simulink model "model_tmp_4p"  (R2015b)
settings: Solver=ode45  StartTime=0.0  StopTime=T_sim  FixedStep=dt  RelTol=1e-3
PreLoadFcn:
  | setup_tmp_4p;
InitFcn:
  | setup_tmp_4p;
StartFcn:
  | setup_tmp_4p;
values from neighbouring files (symbols this model uses):
  A_act = [-100 0 0 0 0 -100 0 0 0 0 -100 0 ... (16 elements, 4x4)]    [CD_spline.mat]    (also in CL_spline.mat; setup.m = -100*eye(4); setup_tmp_1p.m = -100*eye(4); setup_tmp_4p.m = -100*eye(4))
  A_init = [1.0386 0 12.9]    [CD_spline.mat]    (also in CL_spline.mat; setup_KiteModel_4points.m = Pc_init + d_n_r * w_k * w_rel * [-1;0;0])
  A_Kite = 7    [CD_spline.mat]    (also in CL_spline.mat; setup.m = 10.18; setup_tmp_1p.m = 10.18; setup_tmp_4p.m = 10.18)
  A_prd = [0 0 0 -640 0 0 0 0 0 0 -640 0 ... (36 elements, 6x6)]    [CD_spline.mat]    (also in CL_spline.mat; setup.m = 1000 * A_M_aug; setup_tmp_1p.m = 1000 * A_M_aug; setup_tmp_4p.m = 1000 * A_M_aug)
  A_ref = [0 0 0 -10000 0 0 0 0 0 0 -10000 0 ... (36 elements, 6x6)]    [CD_spline.mat]    (also in CL_spline.mat; setup.m = zeros(6); setup_tmp_1p.m = zeros(6); setup_tmp_4p.m = zeros(6))
  A_t_ref_cl = [0 0 0 -0.64 0 0 0 0 0 0 -0.64 0 ... (36 elements, 6x6)]    [CD_spline.mat]    (also in CL_spline.mat; setup.m = A_t_ref; setup_tmp_1p.m = A_t_ref; setup_tmp_4p.m = A_t_ref)
  alpha_0 = 10 * pi/180    (= 0.174532925199)    [setup_KiteModel_4points.m]
  alpha_d_max = 31 * pi/180    (= 0.541052068118)    [setup_KiteModel_4points.m]
  alpha_s_0 = 10 * pi/180    (= 0.174532925199)    [setup_KiteModel_4points.m]
  alpha_s_max = 20 * pi/180    (= 0.349065850399)    [setup_KiteModel_4points.m]
  ASideRel = 0    [CD_spline.mat]    (also in CL_spline.mat; setup.m; setup_tmp_1p.m; setup_tmp_4p.m = 0.306)
  B_act = [100 0 0 0 0 100 0 0 0 0 100 0 ... (16 elements, 4x4)]    [CD_spline.mat]    (also in CL_spline.mat; setup.m = 100*eye(4); setup_tmp_1p.m = 100*eye(4); setup_tmp_4p.m = 100*eye(4))
  B_init = [0 0 15.13]    [CD_spline.mat]    (also in CL_spline.mat; setup_KiteModel_4points.m = Pc_init + h_kite * [0;0;1;])
  B_ref = [0 0 0 10000 0 0 0 0 0 0 10000 0 ... (18 elements, 6x3)]    [CD_spline.mat]    (also in CL_spline.mat; setup.m = zeros(6,3); setup_tmp_1p.m = zeros(6,3); setup_tmp_4p.m = zeros(6,3))
  B_t_ref_cl = [0 0 0 0.64 0 0 0 0 0 0 0.64 0 ... (18 elements, 6x3)]    [CD_spline.mat]    (also in CL_spline.mat)
  Bpbl = [0 0 0 1 0 0 0 0 0 0 1 0 ... (18 elements, 6x3)]    [CD_spline.mat]    (also in CL_spline.mat; setup.m = [zeros(3); eye(3)]; setup_tmp_1p.m = [zeros(3); eye(3)]; setup_tmp_4p.m = [zeros(3); eye(3)])
  c0 = 614000    [CD_spline.mat]    (also in CL_spline.mat; setup.m; setup_tmp_1p.m; setup_tmp_4p.m)
  c_1_TR = 0.262    [setup_KiteModel_4points.m]
  C_A = [0 0.3 -1e-06 1 -0.3 0 1e-06 1 0 -0.3 -1e-06 1 ... (16 elements, 4x4)]    [CD_spline.mat]    (also in CL_spline.mat; setup.m = [0, -R, 0, R; setup_tmp_1p.m = [0, -R, 0, R; setup_tmp_4p.m = [0, -R, 0, R)
  C_A_inv = [0 -1.66666666667 -1.23358113847e-17 1.66666666667 1.66666666667 2.46716227694e-17 -1.66666666667 0 -250000 250000 -250000 250000 ... (16 elements, 4x4)]    [CD_spline.mat]    (also in CL_spline.mat; setup.m = C_A \eye(4); setup_tmp_1p.m = C_A \eye(4); setup_tmp_4p.m = C_A \eye(4))
  C_init = [0 2.5965 12.9]    [CD_spline.mat]    (also in CL_spline.mat; setup_KiteModel_4points.m = Pc_init + 0.5 * w_k * w_rel * [0;1;0])
  CD_spline_coefs = CD_spline.coefs    [setup_KiteModel_4points.m]
  CD_tether = 0.96    [CD_spline.mat]    (also in CL_spline.mat; setup.m; setup_tmp_1p.m; setup_tmp_4p.m)
  CL_spline_coefs = CL_spline.coefs    [setup_KiteModel_4points.m]
  d0 = 473    [CD_spline.mat]    (also in CL_spline.mat; setup.m; setup_tmp_1p.m; setup_tmp_4p.m)
  D_init = [0 -2.5965 12.9]    [CD_spline.mat]    (also in CL_spline.mat; setup_KiteModel_4points.m = Pc_init - 0.5 * w_k * w_rel * [0;1;0])
  d_tether = 0.004    [CD_spline.mat]    (also in CL_spline.mat; setup.m; setup_tmp_1p.m; setup_tmp_4p.m)
  delta_dead = 0.5    [CD_spline.mat]    (also in CL_spline.mat; setup.m; setup_tmp_1p.m; setup_tmp_4p.m)
  e_0 = 0.01    [CD_spline.mat]    (also in CL_spline.mat; setup.m; setup_tmp_1p.m; setup_tmp_4p.m)
  epsilon = 0.6    [CD_spline.mat]    (also in CL_spline.mat; setup.m; setup_tmp_1p.m; setup_tmp_4p.m)
  g = 9.81    [CD_spline.mat]    (also in CL_spline.mat; setup.m; setup_tmp_1p.m; setup_tmp_4p.m)
  g_vec = [0 0 9.81]    [CD_spline.mat]    (also in CL_spline.mat; setup.m = [0;0;9.81]; setup_tmp_1p.m = [0;0;9.81]; setup_tmp_4p.m = [0;0;9.81])
  Gamma_ad = 100    [CD_spline.mat]    (also in CL_spline.mat; setup.m = 100;100; setup_tmp_1p.m = 100;100; setup_tmp_4p.m = 100;100)
  Gamma_pred = 100    [CD_spline.mat]    (also in CL_spline.mat; setup.m; setup_tmp_1p.m; setup_tmp_4p.m)
  J = [0.018  0  0; 0  0.018  0; 0  0  0.009]    [CD_spline.mat]    (also in CL_spline.mat; setup.m = diag([Ixx, Iyy, Izz]); setup_tmp_1p.m = diag([Ixx, Iyy, Izz]); setup_tmp_4p.m = diag([Ixx, Iyy, Izz]))
  Jinv = [55.5555555556  0  0; 0  55.5555555556  0; 0  0  111.111111111]    [CD_spline.mat]    (also in CL_spline.mat; setup.m = J \ eye(3); setup_tmp_1p.m = J \ eye(3); setup_tmp_4p.m = J \ eye(3))
  K = 1 - ASideRel    [setup_KiteModel_4points.m]
  K_d_s = 1.5    [setup_KiteModel_4points.m]
  k_e_eta = 10000    [CD_spline.mat]    (also in CL_spline.mat; setup.m; setup_tmp_1p.m; setup_tmp_4p.m)
  k_e_eta_dot = 400    [CD_spline.mat]    (also in CL_spline.mat; setup.m; setup_tmp_1p.m; setup_tmp_4p.m)
  k_e_eta_I = 1    [CD_spline.mat]    (also in CL_spline.mat; setup.m; setup_tmp_1p.m; setup_tmp_4p.m)
  K_e_psi = 10    [setup_tmp_4p.m]
  K_i_t = [10  0  0; 0  10  0; 0  0  10]    [CD_spline.mat]    (also in CL_spline.mat; setup.m = 10*eye(3); setup_tmp_1p.m = 10*eye(3); setup_tmp_4p.m = 10*eye(3))
  K_v_t = [1.6  0  0; 0  1.6  0; 0  0  1.6]    [CD_spline.mat]    (also in CL_spline.mat; setup.m = 2*omega_0_trans*zeta_0_trans*eye(3); setup_tmp_1p.m = 2*omega_0_trans*zeta_0_trans*eye(3); setup_tmp_4p.m = 2*omega_0_trans*zeta_0_trans*eye(3))
  K_x_t = [0.64  0  0; 0  0.64  0; 0  0  0.64]    [CD_spline.mat]    (also in CL_spline.mat; setup.m = omega_0_trans^2*eye(3); setup_tmp_1p.m = omega_0_trans^2*eye(3); setup_tmp_4p.m = omega_0_trans^2*eye(3))
  l_s0 = 1    [CD_spline.mat]    (also in CL_spline.mat; setup.m = 1.42857142857; setup_tmp_1p.m = 1.42857142857; setup_tmp_4p.m = 2)
  l_s_BP = norm( B_init - p_B_UAV_init)    [setup_KiteModel_4points.m]
  l_s_PUav = norm( pos_UAV_init - p_B_UAV_init)    [setup_KiteModel_4points.m]
  ls_AB = norm( A_init -  B_init)    [setup_KiteModel_4points.m]
  ls_AC = norm( A_init -  C_init)    [setup_KiteModel_4points.m]
  ls_AD = norm( A_init -  D_init)    [setup_KiteModel_4points.m]
  ls_AKcu = norm( A_init -  P_kcu)    [setup_KiteModel_4points.m]
  ls_CB = norm( C_init -  B_init)    [setup_KiteModel_4points.m]
  ls_CD = norm( C_init -  D_init)    [setup_KiteModel_4points.m]
  ls_CKcu = norm( C_init - P_kcu)    [setup_KiteModel_4points.m]
  ls_DB = norm( D_init - B_init )    [setup_KiteModel_4points.m]
  ls_DKcu = norm( D_init - P_kcu)    [setup_KiteModel_4points.m]
  m_A = 3.29    [CD_spline.mat]    (also in CL_spline.mat; setup_KiteModel_4points.m = nose_mass_fraction * m_kite)
  m_B = 1.484    [CD_spline.mat]    (also in CL_spline.mat; setup_KiteModel_4points.m = 0.4 * (1-nose_mass_fraction)*m_kite)
  m_C = 1.113    [CD_spline.mat]    (also in CL_spline.mat; setup_KiteModel_4points.m = 0.3 * (1-nose_mass_fraction)*m_kite)
  m_D = 1.113    [CD_spline.mat]    (also in CL_spline.mat; setup_KiteModel_4points.m = 0.3 * (1-nose_mass_fraction)*m_kite)
  m_kcu = 8.4    [setup_tmp_4p.m]
  m_p = 0.013    [CD_spline.mat]    (also in CL_spline.mat; setup.m = 0.0185714285714; setup_tmp_1p.m = 0.0185714285714; setup_tmp_4p.m = 0.026)
  m_uav = 3    [CD_spline.mat]    (also in CL_spline.mat; setup.m; setup_tmp_1p.m; setup_tmp_4p.m)
  n_t_p = 7    [setup.m]    (also in setup_tmp_1p.m; setup_tmp_4p.m = 5)
  p_B_UAV_init = B_init + [0;0;l_s0]    [setup_KiteModel_4points.m]
  p_init_4p = zeros(3*n_t_p,1)    [setup.m]    (also in setup_tmp_4p.m)
  P_prd = [712.5 0 0 156.25 0 0 0 712.5 0 0 156.25 0 ... (36 elements, 6x6)]    [CD_spline.mat]    (also in CL_spline.mat; setup.m = 1000 * P_tref; setup_tmp_1p.m = 1000 * P_tref; setup_tmp_4p.m = 1000 * P_tref)
  P_tref = [0.7125 0 0 0.15625 0 0 0 0.7125 0 0 0.15625 0 ... (36 elements, 6x6)]    [CD_spline.mat]    (also in CL_spline.mat; setup.m = lyap(A_M_aug', Q); setup_tmp_1p.m = lyap(A_M_aug', Q); setup_tmp_4p.m = lyap(A_M_aug', Q))
  pos_UAV_init = p_B_UAV_init + [0;0;l_s0]    [setup_KiteModel_4points.m]
  rho_air = 1.225    [CD_spline.mat]    (also in CL_spline.mat; setup.m; setup_tmp_1p.m; setup_tmp_4p.m)
  rho_t = 0.013    [CD_spline.mat]    (also in CL_spline.mat; setup.m; setup_tmp_1p.m; setup_tmp_4p.m)
  sample_log = 0.01    [CD_spline.mat]    (also in CL_spline.mat; setup.m; setup_tmp_1p.m; setup_tmp_4p.m)
  T_launch = 40    [CD_spline.mat]    (also in CL_spline.mat; setup.m; setup_tmp_1p.m; setup_tmp_4p.m)
  Theta_max = 60    [CD_spline.mat]    (also in CL_spline.mat; setup.m; setup_tmp_1p.m; setup_tmp_4p.m)
  Thrust_Max = 80    [CD_spline.mat]    (also in CL_spline.mat; setup.m; setup_tmp_1p.m = 100; setup_tmp_4p.m = 1000000000)
  Tx = 10    [CD_spline.mat]    (also in CL_spline.mat; setup.m; setup_tmp_1p.m; setup_tmp_4p.m)
  Ty = 10    [CD_spline.mat]    (also in CL_spline.mat; setup.m; setup_tmp_1p.m; setup_tmp_4p.m)
  Tz = 10    [CD_spline.mat]    (also in CL_spline.mat; setup.m; setup_tmp_1p.m; setup_tmp_4p.m)
  u_d_0 = 0.213    [setup_KiteModel_4points.m]
  u_d_max = 0.47    [setup_KiteModel_4points.m]
  u_s_0 = 0    [setup_KiteModel_4points.m]
  v_w_vec = [1 1 1]    [CD_spline.mat]    (also in CL_spline.mat; setup.m = [1;0;0]; setup_tmp_1p.m = [1;0;0]; setup_tmp_4p.m = [0.01;0;0])
  x0num = 0    [CD_spline.mat]    (also in CL_spline.mat; polynomial_trajectory.m = double( solutions_x.x0 ))
  x1num = 0    [CD_spline.mat]    (also in CL_spline.mat; polynomial_trajectory.m = double( solutions_x.x1 ))
  x2num = 0    [CD_spline.mat]    (also in CL_spline.mat; polynomial_trajectory.m = double( solutions_x.x2 ))
  x3num = 0.05    [CD_spline.mat]    (also in CL_spline.mat; polynomial_trajectory.m = double( solutions_x.x3 ))
  x4num = -0.0075    [CD_spline.mat]    (also in CL_spline.mat; polynomial_trajectory.m = double( solutions_x.x4 ))
  x5num = 0.0003    [CD_spline.mat]    (also in CL_spline.mat; polynomial_trajectory.m = double( solutions_x.x5 ))
  x_drone_init = [0 0 10]    [CD_spline.mat]    (also in CL_spline.mat; setup.m = p_init(3*n-2:3*n); setup_KiteModel_4points.m = pos_UAV_init; setup_tmp_1p.m = p_init(3*n-2:3*n))
  xT = 5    [CD_spline.mat]    (also in CL_spline.mat; setup.m; setup_tmp_1p.m = 10; setup_tmp_4p.m = 10)
  y0num = 0    [CD_spline.mat]    (also in CL_spline.mat; polynomial_trajectory.m = double( solutions_y.y0 ))
  y1num = 0    [CD_spline.mat]    (also in CL_spline.mat; polynomial_trajectory.m = double( solutions_y.y1 ))
  y2num = 0    [CD_spline.mat]    (also in CL_spline.mat; polynomial_trajectory.m = double( solutions_y.y2 ))
  y3num = 0.1    [CD_spline.mat]    (also in CL_spline.mat; polynomial_trajectory.m = double( solutions_y.y3 ))
  y4num = -0.015    [CD_spline.mat]    (also in CL_spline.mat; polynomial_trajectory.m = double( solutions_y.y4 ))
  y5num = 0.0006    [CD_spline.mat]    (also in CL_spline.mat; polynomial_trajectory.m = double( solutions_y.y5 ))
  yT = 10    [CD_spline.mat]    (also in CL_spline.mat; setup.m; setup_tmp_1p.m = 0; setup_tmp_4p.m = 0)
  z0num = 10    [CD_spline.mat]    (also in CL_spline.mat; polynomial_trajectory.m = double( solutions_z.z0 ))
  z1num = 0    [CD_spline.mat]    (also in CL_spline.mat; polynomial_trajectory.m = double( solutions_z.z1 ))
  z2num = 0    [CD_spline.mat]    (also in CL_spline.mat; polynomial_trajectory.m = double( solutions_z.z2 ))
  z3num = 0.4    [CD_spline.mat]    (also in CL_spline.mat; polynomial_trajectory.m = double( solutions_z.z3 ))
  z4num = -0.06    [CD_spline.mat]    (also in CL_spline.mat; polynomial_trajectory.m = double( solutions_z.z4 ))
  z5num = 0.0024    [CD_spline.mat]    (also in CL_spline.mat; polynomial_trajectory.m = double( solutions_z.z5 ))
  zT = 50    [CD_spline.mat]    (also in CL_spline.mat; setup.m; setup_tmp_1p.m; setup_tmp_4p.m)
libraries: simulink x1
(part 3 of 3)

== matlab function model_tmp_4p/Plant/Tether_Kite_Tether_UAV_Dynamics_4P/Tethermodel_Ground2Kite_4P/Tether_Ground2Kite ==
  data: x_dot input; x input; x_dotdot_TetherG2K output; v_w_vec input; d_tether parameter; CD_tether parameter; v_ro_set input; l_s input; c0 parameter; d0 parameter; rho_t parameter; g_vec parameter; rho_air parameter; l_tether output; l_s_dot output; x_kite_A input; x_kite_C input; x_kite_D input; xdot_kite_A input; xdot_kite_C input; xdot_kite_D input; ls_AKcu parameter; ls_CKcu parameter; ls_DKcu parameter; m_kcu parameter
function [x_dotdot_TetherG2K,...
    l_tether, l_s_dot]    = fcn(x_dot, x,  v_w_vec,...
    d_tether, CD_tether, v_ro_set,l_s, c0, d0, rho_t, g_vec, rho_air,...
    x_kite_A,x_kite_C,x_kite_D ,xdot_kite_A,xdot_kite_C,xdot_kite_D, ls_AKcu, ls_CKcu,  ls_DKcu, m_kcu   )

%#codegen
%n = 10;
n_t_p = 5; % amount of groudn particles
l_tether = l_s * n_t_p; % Tether length from ground to kite
l_s_dot = v_ro_set/n_t_p;

% Adapt stiffness and damping with respect to current segment length
c = c0/l_s;
d = d0/l_s;

% Mass of tether segments with  respect to current segment length
m = l_s * rho_t;
m_vec = m * ones(n_t_p,1);
m_vec(n_t_p) = m_kcu;

p_vec = x;
v_vec = x_dot;
p_norm = zeros(n_t_p,1);

% Vector with distances between particles
p_d = p_vec - [0;0;0; p_vec(1:3*n_t_p-3)];

% Vector with velocity differences
v_d = v_vec - [0;0;0; v_vec(1:3*n_t_p-3)];

% calculate absolute distances between points
for iter = 1 : n_t_p
    p_norm(iter) = norm( p_d( (iter-1)* 3 + 1 : (iter-1) * 3 + 3 ) );
end

%%------------------------------- Equations of motions-------------------------------
% Initialize matrices
fsd_tot_mat = zeros(3,n_t_p);
x_dotdot = zeros(3,n_t_p);
D_s_mat = zeros(3,n_t_p);

%% Set up equations of motions of ground to kite tether

% Boundary tether force from kite to particle below kite (in the 4p kite model the kcu is connected to the
% points A, C and D

f_kite_A = calcSpringDamperForce_Bridle( c0,norm( x_kite_A - p_vec(3*(n_t_p) -2 : 3*(n_t_p) ) ), ls_AKcu, d0,...
            x_kite_A - p_vec(3*(n_t_p) -2 : 3*(n_t_p) ) ,...
            xdot_kite_A - v_vec( 3*(n_t_p) -2 : 3*(n_t_p)  ), 1 );
f_kite_C= calcSpringDamperForce_Bridle( c0,norm( x_kite_C - p_vec(3*(n_t_p) -2 : 3*(n_t_p) ) ), ls_CKcu, d0,...
            x_kite_C - p_vec(3*(n_t_p) -2 : 3*(n_t_p) ) ,...
            xdot_kite_C - v_vec( 3*(n_t_p) -2 : 3*(n_t_p) ), 1 );
f_kite_D = calcSpringDamperForce_Bridle( c0,norm( x_kite_D - p_vec(3*(n_t_p) -2 : 3*(n_t_p) ) ), ls_DKcu, d0,...
            x_kite_D - p_vec(3*(n_t_p) -2 : 3*(n_t_p) ) ,...
            xdot_kite_D - v_vec( 3*(n_t_p) -2 : 3*(n_t_p) ), 1 );        
              
for idx = 1 : n_t_p
    
    % Calculate Spring-Damper forces
    fsd_tot_mat(:,idx) = calcSpringDamperForce( c, p_norm(idx), l_s, d, p_d( (idx-1)*3+1:(idx-1)*3+3 ), v_d( (idx-1)*3+1:(idx-1)*3+3), idx );
    if idx < n_t_p
        fsd_tot_mat(:,idx+1) = calcSpringDamperForce( c, p_norm(idx+1), l_s, d, p_d( idx*3+1:idx*3+3 ), v_d( idx*3+1:idx*3+3), idx );       
    end
    
    % Calculate apparent wind speed of tether particles
    if idx == 1 % Segment that is connected to the ground
        v_a_p = v_w_vec - 0.5*x_dot(1:3) ;
    else
        v_a_p = v_w_vec - 0.5*( x_dot((idx-1)*3+1:(idx-1)*3+3) + x_dot((idx-1)*3:(idx-1)*3+2) ); % take mean value of adjacent particle vel. for segment velocity
    end
    
    % Calculate segment drag
    D_s_mat(:,idx) = calcSegmentDrag(p_d((idx-1)*3+1:(idx-1)*3+3) , v_a_p, rho_air, CD_tether, d_tether); % segment drag
    
    if idx < n_t_p
        % Equations of motion for the groud tether particles Newton x_dotdot = 1/m * (-f + u -mg )
        x_dotdot(:,idx) = 1/m_vec(idx) * ( -fsd_tot_mat(:,idx) + fsd_tot_mat(:,idx+1) - m_vec(idx)*g_vec  + D_s_mat(:,idx) );  % Particle dynamics
    else
        x_dotdot(:,idx) = 1/m_vec(idx) * ( -fsd_tot_mat(:,idx) + ...
            f_kite_A + f_kite_C + f_kite_D - m_vec(idx)*g_vec  + D_s_mat(:,idx) );  % Particle dynamics
    end
    
end


%% Reshape the structure of x_dotdot such that x_dotdot = [x1;y1;z1;x2;y2;...]
x_dotdot_TetherG2K = reshape(x_dotdot, [3*n_t_p,1]);

== matlab function model_tmp_4p/Controller/Outer_Loop_Position/Adaptive_Augmentation/Proj(Theta_hat, GammaY)_multicolumns/Projection_Input_2/Proj(Theta,Theta_dot) ==
  data: f input; gradf input; Theta_dot input; Theta_hat_dot_ output
function  Theta_hat_dot_ = fcn(f, gradf, Theta_dot )
%#codegen


if ( f > 0 && gradf*Theta_dot' > 0 )
    Theta_hat_dot_ = Theta_dot - f * ( (gradf'*gradf) / (gradf*gradf') * Theta_dot' )'   ;
else
    Theta_hat_dot_ =  Theta_dot;
end

== matlab function model_tmp_4p/Plant/Tether_Kite_Tether_UAV_Dynamics_4P/UAV_Model/UAV_Dynamics ==
  data: x_dotdot_uav_trans output; omega_dot output; eta_dot output; Thrust input; m_uav parameter; g_vec parameter; x_UAV input; x_below_UAV input; x_dot_UAV input; x_dot_belowUAV input; c0 parameter; d0 parameter; l_s0 parameter; disturbance output; omega input; u_M input; J parameter; Jinv parameter; eta input
function [x_dotdot_uav_trans,omega_dot, eta_dot,  disturbance] = fcn(Thrust, m_uav, g_vec, x_UAV, x_below_UAV, x_dot_UAV, x_dot_belowUAV,...
    c0, d0, l_s0, omega, u_M, J,Jinv,eta )
%#codegen

%% Translational Dynamics
f_T_below = calcSpringDamperForce(c0, norm(x_UAV-x_below_UAV) , l_s0, d0, x_UAV-x_below_UAV, x_dot_UAV - x_dot_belowUAV, 1 );
disturbance = -f_T_below/m_uav;
%disturbance = 1/m_uav *[0;0;25] ;
x_dotdot_uav_trans = 1/m_uav * ( -0*f_T_below + Thrust - m_uav*g_vec + 0*[0;0;25]  ) ; % Drone dynamics

%% Rotational Dynamics 
p = omega(1); 
q = omega(2); 
r = omega(3); 
Ix = J(1,1); 
Iy = J(2,2); 
Iz = J(3,3); 

cross_coupling = [ Iy*q*r - Iz*q*r
                   Iz*p*r - Ix*p*r;
                   Ix*p*q - Iy*p*q];
% Bodyrate Dynamics
omega_dot = Jinv * ( cross_coupling + u_M ) ;  

% Attitude Dynamics
eta_dot = [1, sin(eta(1)) * tan(eta(2)), cos(eta(1)) * tan(eta(2)) ; 
0, cos(eta(1)), -sin(eta(1)); 
0, sin(eta(1))/cos(eta(2)), cos(eta(1))/cos(eta(2))] * omega ;

== matlab function model_tmp_4p/Controller/Outer_Loop_Position/Adaptive_Augmentation/Proj(Theta_hat, GammaY)_multicolumns/Projection_Input_2/calculate_f ==
  data: theta_hat input; f output; Theta_max input; epsilon input
function f   = fcn(theta_hat,Theta_max, epsilon )
%#codegen
f = ( (1+epsilon)*norm(theta_hat)^2 - (Theta_max)^2 ) / (epsilon*(Theta_max)^2);

== matlab function model_tmp_4p/Controller/Outer_Loop_Position/Adaptive_Augmentation/Proj(Theta_hat, GammaY)_multicolumns/Projection_Input_2/calculate_gradf ==
  data: theta_hat input; gradf output; Theta_max input; epsilon input
function gradf = fcn(theta_hat,Theta_max, epsilon )
%#codegen
gradf = ( 2*(1+epsilon) ) / (epsilon*(Theta_max)^2) * theta_hat ;

== matlab function model_tmp_4p/Controller/Outer_Loop_Position/Adaptive_Augmentation/Proj(Theta_hat, GammaY)_multicolumns/Projection_Input_3/Proj(Theta,Theta_dot) ==
  data: flag output; f input; gradf input; Theta_dot input; Theta_hat_dot_ output; direction output
function  [flag,Theta_hat_dot_, direction] = fcn(f, gradf, Theta_dot )
%#codegen


if ( f > 0 && gradf*Theta_dot' > 0 )
    flag  = 1;
    direction = gradf*Theta_dot';
    Theta_hat_dot_ = Theta_dot - f * ( (gradf'*gradf) / (gradf*gradf') * Theta_dot' )'   ;
else
    direction = gradf*Theta_dot';
    flag = 0;
    Theta_hat_dot_ =  Theta_dot;
end

== matlab function model_tmp_4p/Controller/Outer_Loop_Position/Adaptive_Augmentation/Proj(Theta_hat, GammaY)_multicolumns/Projection_Input_3/calculate_f ==
  data: theta_hat input; f output; Theta_max input; epsilon input
function f   = fcn(theta_hat,Theta_max, epsilon )
%#codegen
f = ( (1+epsilon)*norm(theta_hat)^2 - (Theta_max)^2 ) / (epsilon*(Theta_max)^2);

== matlab function model_tmp_4p/Controller/Outer_Loop_Position/Adaptive_Augmentation/Proj(Theta_hat, GammaY)_multicolumns/Projection_Input_3/calculate_gradf ==
  data: theta_hat input; gradf output; Theta_max input; epsilon input
function gradf = fcn(theta_hat,Theta_max, epsilon )
%#codegen
gradf = ( 2*(1+epsilon) ) / (epsilon*(Theta_max)^2) * theta_hat ;

== matlab function model_tmp_4p/Controller/Inner_Loop_Attitude/Reference_Model1/Reference Model 2nd order ==
  data: eta_c input; eta_r_dot output; A_r input; B_r input; eta_r_dotdot output; x input
function [eta_r_dot, eta_r_dotdot] = fcn(eta_c, A_r, B_r, x)


x_dot = A_r * x + B_r * eta_c;

eta_r_dot = x_dot(1:3);
eta_r_dotdot = x_dot(4:6);
